simulink model "HAPSRAV_ENERGY_OPT"  (R2017a)
settings: Solver=ode1  StartTime=0.0  StopTime=tfin  FixedStep=dT  MaxStep=dT*10  MinStep=dT  RelTol=1e-3
libraries: hapsrav_library x2
settings Model: SimulationMode=accelerator  Creator=jack.marriott  LastModifiedBy=marriott
settings SolverCC: InitialStep=dT  ZeroCrossControl=EnableAll
settings DataIOCC: SaveOutput=off  SignalLogging=off  DSMLogging=off  ReturnWorkspaceOutputs=on  ReturnWorkspaceOutputsName=ksim
settings OptimizationCC: DefaultParameterBehavior=Inlined  InlineInvariantSignals=on
settings DebuggingCC: RTPrefix=none  ReadBeforeWriteMsg=DisableAll  WriteAfterWriteMsg=DisableAll  WriteAfterReadMsg=DisableAll  MultiTaskDSMMsg=none
settings HardwareCC: TargetBitPerPointer=64  TargetBitPerSizeT=64  TargetBitPerPtrDiffT=64  TargetLongLongMode=on  TargetIntDivRoundTo=Zero  TargetEndianess=LittleEndian  TargetWordSize=64  TargetHWDeviceType=MATLAB Host  ProdEqTarget=off
settings ModelReferenceCC: UpdateModelReferenceTargets=IfOutOfDate
settings SFSimCC: SimUserSources=date_vec.c  SFSimEcho=off
settings RTWCC: SystemTargetFile=rsim.tlc  TemplateMakefile=rsim_default_tmf  Description=Rapid Simulation Target  RTWUseSimCustomCode=on  CustomSource=date_vec.c
settings TargetCC: TargetLangStandard=C99 (ISO)  ParMdlRefBuildCompliant=on  ConcurrentExecutionCompliant=on  GeneratePreprocessorConditionals=Use local settings  MatFileLogging=on  SupportNonFinite=off

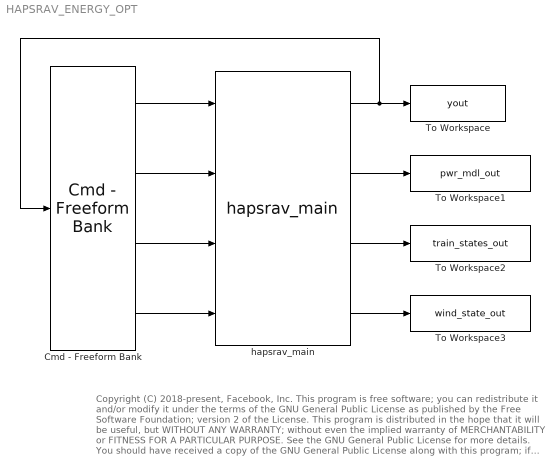
== system HAPSRAV_ENERGY_OPT ==
  note: Copyright (C) 2018-present, Facebook, Inc.
      |
      | This program is free software; you can redistribute it and/or modify
      | it under the terms of the GNU General Public License as published by
      | the Free Software Foundation; version 2 of the License.
      |
      | This program is distributed in the hope that it will be useful,
      | but WITHOUT ANY WARRANTY; without even the implied warranty of
      | MERCHANTABILITY or FITNESS FOR A PARTICULAR PURPOSE. See the
      | GNU General Public License for more details.
      |
      | You should have received a copy of the GNU General Public License along
      | with this program; if not, write to the Free Software Foundation, Inc.,
      | 51 Franklin Street, Fifth Floor, Boston, MA 02110-1301 USA. PATENTS file in the same directory.
  Cmd - Freeform Bank : hapsrav_library/Cmd - Freeform Bank
  To Workspace : ToWorkspace  VariableName=yout  SaveFormat=Structure  SampleTime=-1
  To Workspace1 : ToWorkspace  VariableName=pwr_mdl_out  SaveFormat=Structure  SampleTime=-1
  To Workspace2 : ToWorkspace  VariableName=train_states_out  SaveFormat=Structure  SampleTime=-1
  To Workspace3 : ToWorkspace  VariableName=wind_state_out  SaveFormat=Structure  SampleTime=-1
  hapsrav_main : hapsrav_library/hapsrav_main
  wires:
  Cmd - Freeform Bank/1 -> hapsrav_main/1
  Cmd - Freeform Bank/2 -> hapsrav_main/2
  Cmd - Freeform Bank/3 -> hapsrav_main/3
  Cmd - Freeform Bank/4 -> hapsrav_main/4
  hapsrav_main/2 -> To Workspace1/1
  hapsrav_main/3 -> To Workspace2/1
  hapsrav_main/4 -> To Workspace3/1
  hapsrav_main/1 -> Cmd - Freeform Bank/1, To Workspace/1
